simulink model "feedforward"  (R2019a)
settings: Solver=ode2  StartTime=0.0  StopTime=300  FixedStep=0.1  RelTol=1e-3
settings Model: Creator=HP  LastModifiedBy=swastik
settings DataIOCC: ReturnWorkspaceOutputs=off
settings DebuggingCC: ArithmeticOperatorsInVariantConditions=warning

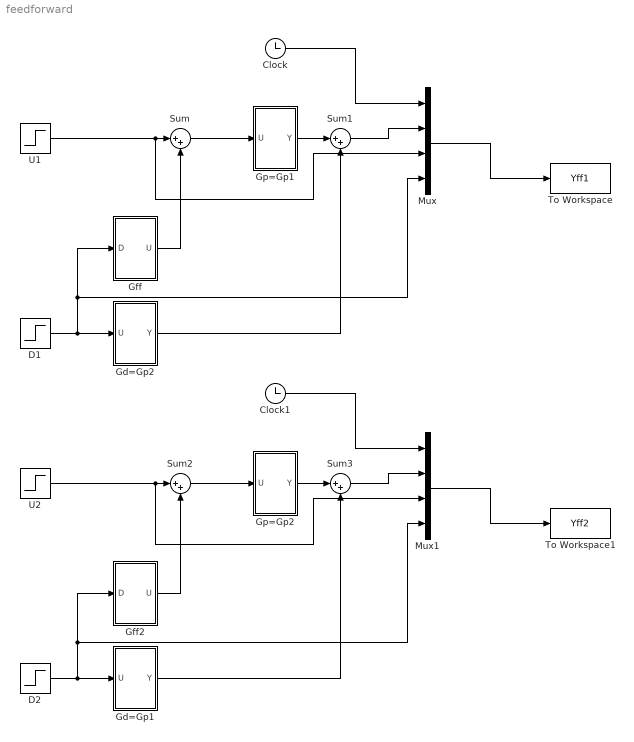
== system feedforward ==
  Clock : Clock
  Clock1 : Clock
  D1 : Step  Time=0  SampleTime=0
  D2 : Step  Time=0  SampleTime=0
  Gd=Gp1 : Subsystem  mask{K=1.9886, T=17.4, D=14}
      mask prompts: K "Gain"; T "Lag Time"; D "Dead Time"
  Gd=Gp2 : Subsystem  mask{K2=0.9894, T2=26.1, D2=20.6}
      mask prompts: K2 "Gain"; T2 "Lag time"; D2 "Dead Time"
  Gff : Subsystem
  Gff2 : Subsystem
  Gp=Gp1 : Subsystem  mask{K=1.9886, T=17.4, D=14}
      mask prompts: K "Gain"; T "Lag Time"; D "Dead Time"
  Gp=Gp2 : Subsystem  mask{K2=0.9894, T2=26.1, D2=20.6}
      mask prompts: K2 "Gain"; T2 "Lag time"; D2 "Dead Time"
  Mux : Mux
  Mux1 : Mux
  Sum{,1..3} (4 alike) : Sum  Inputs=|++
  To Workspace : ToWorkspace  VariableName=Yff1  SampleTime=-1
  To Workspace1 : ToWorkspace  VariableName=Yff2  SampleTime=-1
  U1 : Step  Time=0  SampleTime=0
  U2 : Step  Time=0  SampleTime=0
  wires:
  Clock/1 -> Mux/1
  Mux/1 -> To Workspace/1
  D1/1 -> Gd=Gp2/1(U), Gff/1(D), Mux/4
  U1/1 -> Mux/3, Sum/1
  Gff/1(U) -> Sum/2
  Sum/1 -> Gp=Gp1/1(U)
  Gp=Gp1/1(Y) -> Sum1/1
  Gd=Gp2/1(Y) -> Sum1/2
  Sum1/1 -> Mux/2
  Gp=Gp2/1(Y) -> Sum3/1
  Sum2/1 -> Gp=Gp2/1(U)
  Gd=Gp1/1(Y) -> Sum3/2
  Gff2/1(U) -> Sum2/2
  Mux1/1 -> To Workspace1/1
  U2/1 -> Mux1/3, Sum2/1
  Sum3/1 -> Mux1/2
  Clock1/1 -> Mux1/1
  D2/1 -> Gd=Gp1/1(U), Gff2/1(D), Mux1/4

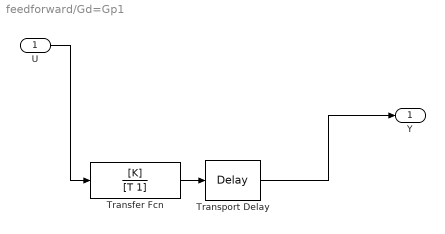
== system feedforward/Gd=Gp1 ==
  U : Inport
  Transfer Fcn : TransferFcn  Numerator=[K]  Denominator=[T 1]
  Transport Delay : TransportDelay  DelayTime=D
  Y : Outport
  wires:
  Transfer Fcn/1 -> Transport Delay/1
  U/1 -> Transfer Fcn/1
  Transport Delay/1 -> Y/1

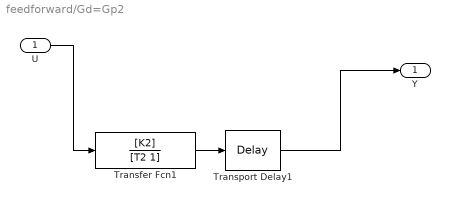
== system feedforward/Gd=Gp2 ==
  U : Inport
  Transfer Fcn1 : TransferFcn  Numerator=[K2]  Denominator=[T2 1]
  Transport Delay1 : TransportDelay  DelayTime=D2
  Y : Outport
  wires:
  Transfer Fcn1/1 -> Transport Delay1/1
  Transport Delay1/1 -> Y/1
  U/1 -> Transfer Fcn1/1

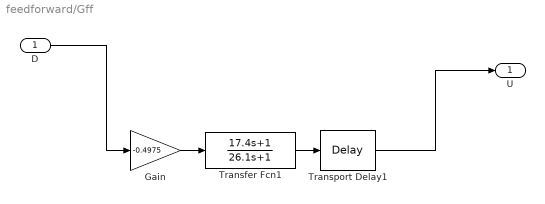
== system feedforward/Gff ==
  D : Inport
  Gain : Gain  Gain=-0.4975
  Transfer Fcn1 : TransferFcn  Numerator=[17.4 1]  Denominator=[26.1 1]
  Transport Delay1 : TransportDelay  DelayTime=20.6-14
  U : Outport
  wires:
  Transfer Fcn1/1 -> Transport Delay1/1
  Transport Delay1/1 -> U/1
  Gain/1 -> Transfer Fcn1/1
  D/1 -> Gain/1

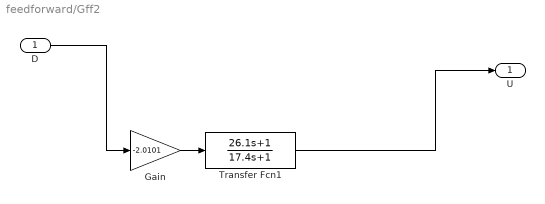
== system feedforward/Gff2 ==
  D : Inport
  Gain : Gain  Gain=-2.0101
  Transfer Fcn1 : TransferFcn  Numerator=[26.1 1]  Denominator=[17.4 1]
  U : Outport
  wires:
  Transfer Fcn1/1 -> U/1
  Gain/1 -> Transfer Fcn1/1
  D/1 -> Gain/1

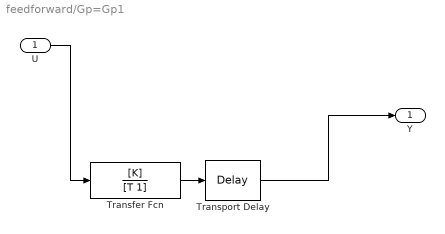
== system feedforward/Gp=Gp1 ==
  U : Inport
  Transfer Fcn : TransferFcn  Numerator=[K]  Denominator=[T 1]
  Transport Delay : TransportDelay  DelayTime=D
  Y : Outport
  wires:
  Transfer Fcn/1 -> Transport Delay/1
  U/1 -> Transfer Fcn/1
  Transport Delay/1 -> Y/1

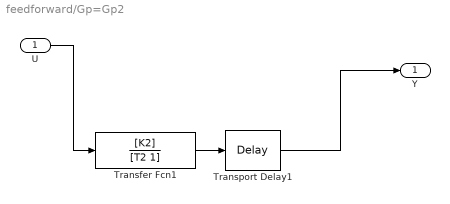
== system feedforward/Gp=Gp2 ==
  U : Inport
  Transfer Fcn1 : TransferFcn  Numerator=[K2]  Denominator=[T2 1]
  Transport Delay1 : TransportDelay  DelayTime=D2
  Y : Outport
  wires:
  Transfer Fcn1/1 -> Transport Delay1/1
  Transport Delay1/1 -> Y/1
  U/1 -> Transfer Fcn1/1
